simulink model "L5z1"  (R2017a)
settings: Solver=VariableStepAuto  StartTime=0.0  StopTime=16  RelTol=1e-3
settings Model: Creator=DoktorHax  LastModifiedBy=DoktorHax

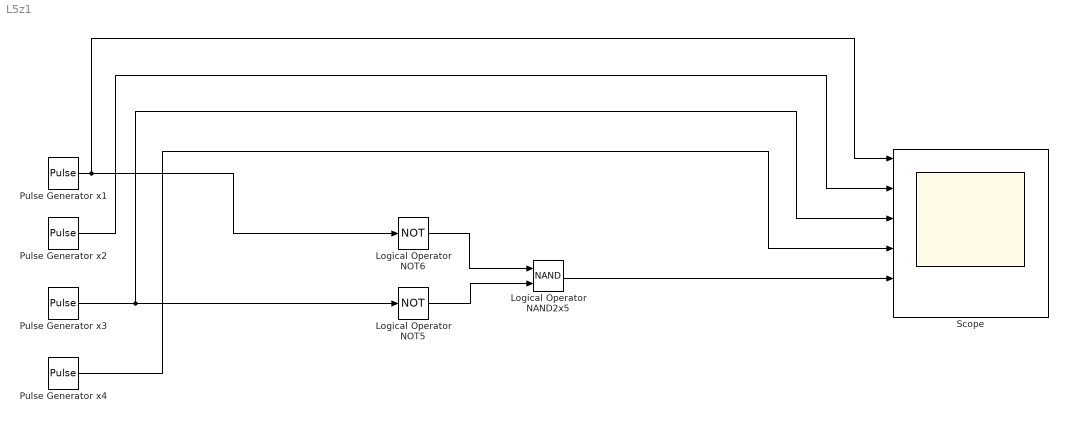
== system L5z1 ==
  Logical Operator NAND2x5 : Logic  Operator=NAND  AllPortsSameDT=off  OutDataTypeStr=boolean
  Logical Operator NOT5 : Logic  Operator=NOT  AllPortsSameDT=off  OutDataTypeStr=boolean
  Logical Operator NOT6 : Logic  Operator=NOT  AllPortsSameDT=off  OutDataTypeStr=boolean
  Pulse Generator x1 : DiscretePulseGenerator  PulseType=Time based  PulseWidth=50
  Pulse Generator x2 : DiscretePulseGenerator  PulseType=Time based  Period=4  PulseWidth=50
  Pulse Generator x3 : DiscretePulseGenerator  PulseType=Time based  Period=8  PulseWidth=50
  Pulse Generator x4 : DiscretePulseGenerator  PulseType=Time based  Period=16  PulseWidth=50
  Scope : Scope  NumInputPorts=6
  wires:
  Pulse Generator x2/1 -> Scope/2
  Pulse Generator x4/1 -> Scope/4
  Pulse Generator x3/1 -> Logical Operator NOT5/1, Scope/3
  Pulse Generator x1/1 -> Scope/1, Logical Operator NOT6/1
  Logical Operator NOT6/1 -> Logical Operator NAND2x5/1
  Logical Operator NOT5/1 -> Logical Operator NAND2x5/2
  Logical Operator NAND2x5/1 -> Scope/5
